simulink model "MpptControl"  (R2020b)
settings: Solver=FixedStepDiscrete  StartTime=0.0  StopTime=10.0  RelTol=1e-3
settings Model: DataDictionary=objDict.sldd  Creator=on4ip  LastModifiedBy=on4ip
settings OptimizationCC: DefaultParameterBehavior=Inlined  UseDivisionForNetSlopeComputation=on  GainParamInheritBuiltInType=on  UseFloatMulNetSlope=on  InlineInvariantSignals=on  EnhancedBackFolding=on  PassReuseOutputArgsAs=Individual arguments  ZeroExternalMemoryAtStartup=off  ZeroInternalMemoryAtStartup=off  NoFixptDivByZeroProtection=on  EfficientFloat2IntCast=on  LifeSpan=1  OptimizeBlockOrder=speed  DifferentSizesBufferReuse=on  LabelGuidedReuse=on  EfficientTunableParamExpr=on
settings DebuggingCC: ParameterTunabilityLossMsg=error
settings HardwareCC: ProdBitPerInt=16  ProdBitPerPointer=16  ProdBitPerSizeT=16  ProdBitPerPtrDiffT=16  ProdLargestAtomicFloat=None  ProdWordSize=16  ProdLongLongMode=on  ProdHWDeviceType=STMicroelectronics->ST10/Super10
settings ModelReferenceCC: ModelReferenceNumInstancesAllowed=Single
settings SFSimCC: MATLABDynamicMemAlloc=off
settings RTWCC: Description=Embedded Coder  SystemTargetFile=ert.tlc  GenCodeOnly=on  TemplateMakefile=ert_default_tmf  GenerateReport=on  GenerateCodeMetricsReport=on
settings CodeAppCC: ForceParamTrailComments=on  IgnoreCustomStorageClasses=off  OperatorAnnotations=on  SimulinkDataObjDesc=on  SFDataObjDesc=on  CustomSymbolStrGlobalVar=$N$M  CustomSymbolStrType=$N$M  CustomSymbolStrFcn=$N$M$F  CustomSymbolStrFcnArg=$N$M  CustomSymbolStrBlkIO=local_$N$M  CustomSymbolStrMacro=$N$M  InsertBlockDesc=on
settings ERTTargetCC: TargetLangStandard=C99 (ISO)  GenerateSampleERTMain=on  IncludeMdlTerminateFcn=off  CombineSignalStateStructs=on  SuppressErrorStatus=on  SupportAbsoluteTime=off  SupportNonFinite=off  SupportComplex=off  SupportNonInlinedSFcns=on  InlinedParameterPlacement=NonHierarchical  MultiInstanceErrorCode=None  ERTCustomFileTemplate=example_file_process.tlc

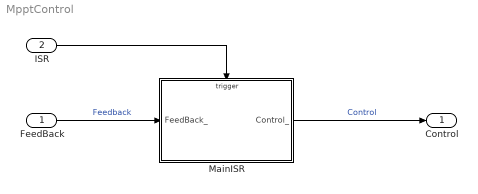
== system MpptControl ==
  FeedBack : Inport  OutDataTypeStr=Bus: FeedBack_st  BusOutputAsStruct=on
  ISR : Inport  Port=2  OutputFunctionCall=on
  MainISR : Subsystem  TreatAsAtomicUnit=on
      settings: FunctionInterfaceSpec=Allow arguments (Optimized)
  Control : Outport  OutDataTypeStr=Bus: Control_st  BusOutputAsStruct=on
  wires:
  FeedBack/1 -> MainISR/1(FeedBack_)  "Feedback"
  MainISR/1(Control_) -> Control/1  "Control"
  ISR/1 -> MainISR/Trigger

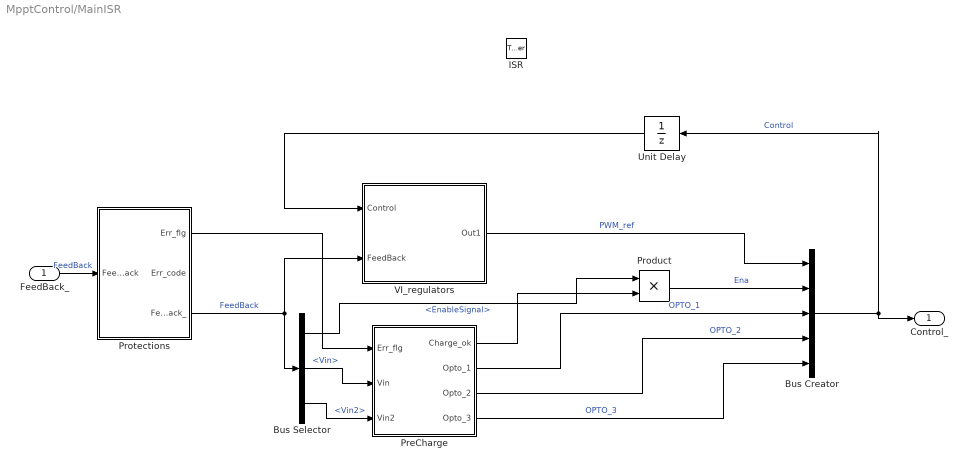
== system MpptControl/MainISR ==
  FeedBack_ : Inport
  ISR : TriggerPort  TriggerType=function-call  VariantControl=Variant  PortDimensions=1
  Bus Creator : BusCreator  Inputs=5  OutDataTypeStr=Bus: Control_st  NonVirtualBus=on
  Bus Selector : BusSelector  OutputSignals=EnableSignal,Vin,Vin2
  PreCharge : Stateflow chart  TreatAsAtomicUnit=on
      settings: RTWSystemCode=Nonreusable function  FunctionInterfaceSpec=Allow arguments (Optimized)
  Product : Product  OutDataTypeStr=Inherit: Inherit via back propagation
  Protections : Subsystem
  Unit Delay : UnitDelay  SampleTime=-1  HasFrameUpgradeWarning=on
  VI_regulators : Subsystem  TreatAsAtomicUnit=on
      settings: MinAlgLoopOccurrences=on
  Control_ : Outport
  wires:
  PreCharge/2(Opto_1) -> Bus Creator/3  "OPTO_1"
  Product/1 -> Bus Creator/2  "Ena"
  PreCharge/4(Opto_3) -> Bus Creator/5  "OPTO_3"
  Bus Creator/1 -> Unit Delay/1, Control_/1  "Control"
  PreCharge/3(Opto_2) -> Bus Creator/4  "OPTO_2"
  Protections/3(FeedBack_) -> Bus Selector/1, VI_regulators/2(FeedBack)  "FeedBack"
  VI_regulators/1(Out1) -> Bus Creator/1  "PWM_ref"
  Unit Delay/1 -> VI_regulators/1(Control)
  Bus Selector/2 -> PreCharge/2(Vin)  "<Vin>"
  Bus Selector/3 -> PreCharge/3(Vin2)  "<Vin2>"
  Bus Selector/1 -> Product/1  "<EnableSignal>"
  PreCharge/1(Charge_ok) -> Product/2
  FeedBack_/1 -> Protections/1(FeedBack)  "FeedBack"
  Protections/1(Err_flg) -> PreCharge/1(Err_flg)

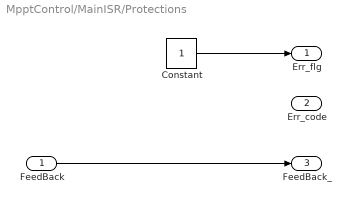
== system MpptControl/MainISR/Protections ==
  FeedBack : Inport
  Constant : Constant  OutDataTypeStr=uint16  SampleTime=-1
  Err_flg : Outport
  Err_code : Outport  Port=2
  FeedBack_ : Outport  Port=3
  wires:
  FeedBack/1 -> FeedBack_/1
  Constant/1 -> Err_flg/1

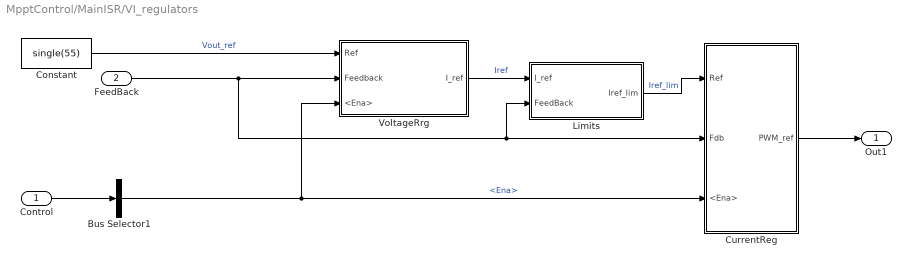
== system MpptControl/MainISR/VI_regulators ==
  Control : Inport
  FeedBack : Inport  Port=2
  Bus Selector1 : BusSelector  OutputSignals=Ena
  Constant : Constant  Value=single(55)
  CurrentReg : Subsystem
  Limits : Subsystem
  VoltageRrg : Subsystem
  Out1 : Outport
  wires:
  Control/1 -> Bus Selector1/1
  Bus Selector1/1 -> VoltageRrg/3(<Ena>), CurrentReg/3(<Ena>)  "<Ena>"
  Constant/1 -> VoltageRrg/1(Ref)  "Vout_ref"
  FeedBack/1 -> Limits/2(FeedBack), CurrentReg/2(Fdb), VoltageRrg/2(Feedback)
  VoltageRrg/1(I_ref) -> Limits/1(I_ref)  "Iref"
  CurrentReg/1(PWM_ref) -> Out1/1
  Limits/1(Iref_lim) -> CurrentReg/1(Ref)  "Iref_lim"

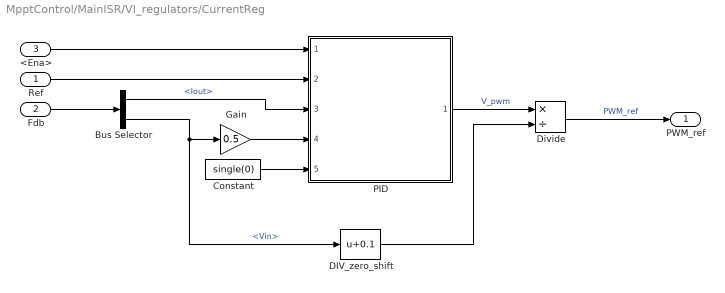
== system MpptControl/MainISR/VI_regulators/CurrentReg ==
  Ref : Inport
  Fdb : Inport  Port=2
  <Ena> : Inport  Port=3
  Bus Selector : BusSelector  OutputSignals=Iout,Vin
  Constant : Constant  Value=single(0)
  DIV_zero_shift : Bias  Bias=0.1
  Divide : Product  Inputs=*/
  Gain : Gain  Gain=0.5
  PID : Subsystem  TreatAsAtomicUnit=on  ReferencedSubsystem=PID_  Kp=0.8  Ki=0.075  Kc=0.9  High=60  Low=0
      settings: MinAlgLoopOccurrences=on  RTWFcnNameOpts=Use subsystem name  RTWFileNameOpts=Use function name  FunctionInterfaceSpec=Allow arguments (Optimized)
  PWM_ref : Outport
  wires:
  DIV_zero_shift/1 -> Divide/2
  <Ena>/1 -> PID/1
  Divide/1 -> PWM_ref/1  "PWM_ref"
  PID/1 -> Divide/1  "V_pwm"
  Ref/1 -> PID/2
  Fdb/1 -> Bus Selector/1
  Bus Selector/2 -> Gain/1, DIV_zero_shift/1  "<Vin>"
  Constant/1 -> PID/5
  Bus Selector/1 -> PID/3  "<Iout>"
  Gain/1 -> PID/4

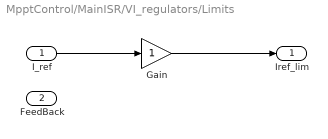
== system MpptControl/MainISR/VI_regulators/Limits ==
  I_ref : Inport
  FeedBack : Inport  Port=2
  Gain : Gain
  Iref_lim : Outport
  wires:
  I_ref/1 -> Gain/1
  Gain/1 -> Iref_lim/1

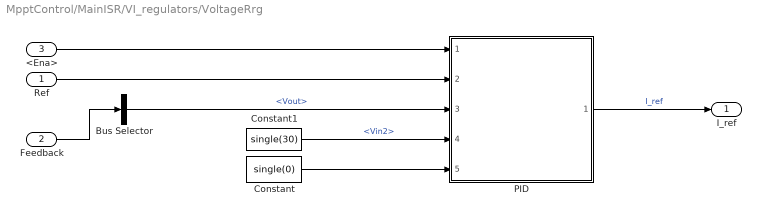
== system MpptControl/MainISR/VI_regulators/VoltageRrg ==
  Ref : Inport
  Feedback : Inport  Port=2
  <Ena> : Inport  Port=3
  Bus Selector : BusSelector  OutputSignals=Vout
  Constant : Constant  Value=single(0)
  Constant1 : Constant  Value=single(30)
  PID : Subsystem  TreatAsAtomicUnit=on  ReferencedSubsystem=PID_  Kp=1.8  Ki=0.075  Kc=0.9  High=60  Low=0
      settings: MinAlgLoopOccurrences=on  RTWFcnNameOpts=Use subsystem name  RTWFileNameOpts=Use function name  FunctionInterfaceSpec=Allow arguments (Optimized)
  I_ref : Outport
  wires:
  Bus Selector/1 -> PID/3  "<Vout>"
  <Ena>/1 -> PID/1
  Constant1/1 -> PID/4  "<Vin2>"
  Constant/1 -> PID/5
  Ref/1 -> PID/2
  PID/1 -> I_ref/1  "I_ref"
  Feedback/1 -> Bus Selector/1

== stateflow chart MpptControl/MainISR/PreCharge ==
  state WORK_MODE
    state START
      entry:
      Opto_1=0;
      Opto_2=0;
      Opto_3=0;
      Charge_ok=0;
      Wait_cnt=0;
      Wait_trashold=2000;
    state PRECARGE_START
      entry:
      Opto_3=1;
      during:
      Wait_cnt = uint16(temporalCount(tick)) ;
    state PRECHARGE_END
      entry:
      Opto_1=1;
      Opto_2=1;
      Charge_ok=1;
    state PRECHARGE_FAIL
      entry:
      Charge_fail=1;
      Charge_ok=0;
    (default) -> START
    START -> PRECARGE_START : [Vin2>VoltageLevel]
    PRECARGE_START -> PRECHARGE_FAIL [order 2] : [Wait_trashold < Wait_cnt]
    PRECARGE_START -> PRECHARGE_END [order 1] : [(Vin2-Vin)<2.1]
  state ERROR_MODE
    entry:
    Opto_1=0;
    Opto_2=0;
    Opto_3=0;
    Charge_ok=0;
    Wait_cnt=0;
    Wait_trashold=2000;
  (default) -> ERROR_MODE
  ERROR_MODE -> WORK_MODE : [~Err_flg]
  WORK_MODE -> ERROR_MODE : [Err_flg]
  data: Err_flg input; Charge_ok output uint16; Vin input; Vin2 input; Opto_1 output uint16; Opto_2 output uint16; Opto_3 output uint16; VoltageLevel constant single; Wait_cnt local uint16; Charge_fail local uint16; Wait_trashold local
